simulink subsystem "Bandwidth_Check_Between_Two_Points"  (R2023b)
settings: Solver=VariableStepAuto  StartTime=0.0  StopTime=10.0  RelTol=1e-3
libraries: simulink x2
settings Model: Creator=FIRSTMentor  LastModifiedBy=ander

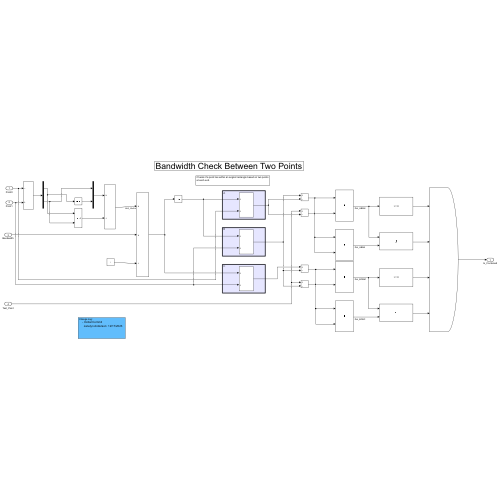
[thumbnail: Simulink's stored preview of the top-level diagram]
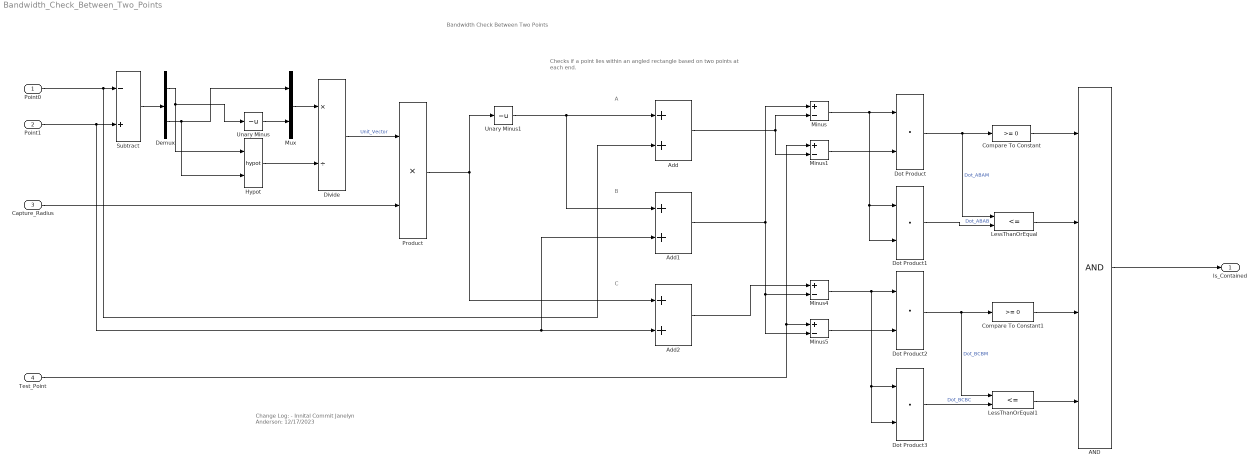
== system Bandwidth_Check_Between_Two_Points ==
  note: A
  note: B
  note: C
  note: Bandwidth Check Between Two Points
  note: Checks if a point lies within an angled rectangle based on two points at each end.
  note: Change Log:
      | - Innital Commit
      | Janelyn Anderson: 12/17/2023
  Point0 : Inport  Unit=m  PortDimensions=[1 2]
  Point1 : Inport  Port=2  Unit=m  PortDimensions=[1 2]
  Capture_Radius : Inport  Port=3  PortDimensions=1
  Test_Point : Inport  Port=4  Unit=m  PortDimensions=[1 2]
  AND : Logic  Inputs=4  AllPortsSameDT=off  OutDataTypeStr=boolean
  Add : Sum
  Add1 : Sum
  Add2 : Sum
  Compare To Constant : simulink/Logic and Bit Operations/Compare To Constant  relop=>=  const=0  OutDataTypeStr=boolean
  Compare To Constant1 : simulink/Logic and Bit Operations/Compare To Constant  relop=>=  const=0  OutDataTypeStr=boolean
  Demux : Demux  Outputs=2
  Divide : Product  Inputs=*/
  Dot Product{,1..3} (4 alike) : DotProduct  OutDataTypeStr=Inherit: Inherit via internal rule
  Hypot : Math  Operator=hypot
  LessThanOrEqual : RelationalOperator  Operator=<=  OutDataTypeStr=boolean  RndMeth=Simplest  InputSameDT=off
  LessThanOrEqual1 : RelationalOperator  Operator=<=  OutDataTypeStr=boolean  RndMeth=Simplest  InputSameDT=off
  Minus{,1,4..5} (4 alike) : Sum  Inputs=+-
  Mux : Mux  Inputs=2
  Product : Product  Inputs=**
  Subtract : Sum  Inputs=-+
  Unary Minus : UnaryMinus
  Unary Minus1 : UnaryMinus
  Is_Contained : Outport
  wires:
  Dot Product3/1 -> LessThanOrEqual1/2  "Dot_BCBC"
  Add1/1 -> Minus5/2, Minus4/2, Minus/1
  Minus/1 -> Dot Product/1, Dot Product1/2, Dot Product1/1
  Dot Product/1 -> LessThanOrEqual/1, Compare To Constant/1  "Dot_ABAM"
  Mux/1 -> Divide/1
  Minus1/1 -> Dot Product/2
  Divide/1 -> Product/1  "Unit_Vector"
  Demux/1 -> Hypot/1, Unary Minus/1
  Subtract/1 -> Demux/1
  Hypot/1 -> Divide/2
  Point1/1 -> Subtract/2, Add1/2, Add2/2
  Demux/2 -> Hypot/2, Mux/1
  Unary Minus1/1 -> Add1/1, Add/1
  Minus5/1 -> Dot Product2/2
  Product/1 -> Unary Minus1/1, Add2/1
  Compare To Constant/1 -> AND/1
  AND/1 -> Is_Contained/1
  LessThanOrEqual1/1 -> AND/4
  Dot Product1/1 -> LessThanOrEqual/2  "Dot_ABAB"
  LessThanOrEqual/1 -> AND/2
  Dot Product2/1 -> Compare To Constant1/1, LessThanOrEqual1/1  "Dot_BCBM"
  Compare To Constant1/1 -> AND/3
  Minus4/1 -> Dot Product2/1, Dot Product3/1, Dot Product3/2
  Point0/1 -> Add/2, Subtract/1
  Add/1 -> Minus1/2, Minus/2
  Capture_Radius/1 -> Product/2
  Add2/1 -> Minus4/1
  Test_Point/1 -> Minus1/1, Minus5/1
  Unary Minus/1 -> Mux/2
